simulink model "half_bridge"  (R2020a)
settings: Solver=VariableStepAuto  StartTime=0.0  StopTime=0.005  RelTol=1e-3
libraries: powerlib x25
settings Model: Creator=tomi_  LastModifiedBy=tomi_

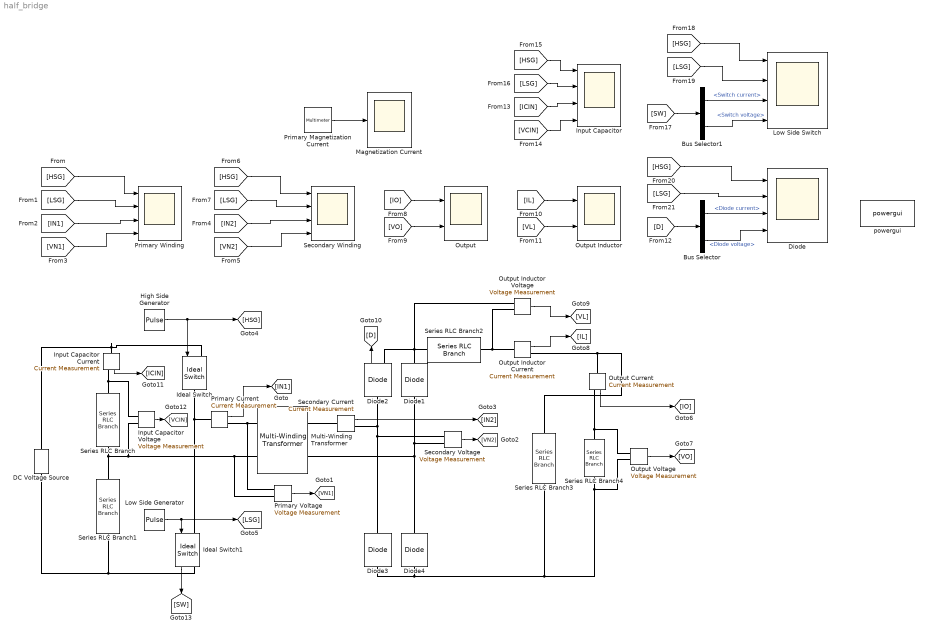
== system half_bridge ==
  Bus Selector : BusSelector  OutputSignals=Diode current,Diode voltage
  Bus Selector1 : BusSelector  OutputSignals=Switch current,Switch voltage
  DC Voltage Source : powerlib/Electrical Sources/DC Voltage Source  Amplitude=13.8  Measurements=None
  Diode : Scope  NumInputPorts=4
  Diode1 : powerlib/Power Electronics/Diode  Ron=0.0001  Lon=0  Vf=1  IC=0  UseSnubber=0  Rs=10e6  Cs=0  Measurements=off
  Diode2 : powerlib/Power Electronics/Diode  Ron=0.0001  Lon=0  Vf=1  IC=0  UseSnubber=0  Rs=10e6  Cs=0  Measurements=on
  Diode3 : powerlib/Power Electronics/Diode  Ron=0.0001  Lon=0  Vf=1  IC=0  UseSnubber=0  Rs=10e6  Cs=0  Measurements=off
  Diode4 : powerlib/Power Electronics/Diode  Ron=0.0001  Lon=0  Vf=1  IC=0  UseSnubber=0  Rs=10e6  Cs=0  Measurements=off
  High Side Generator : DiscretePulseGenerator  PulseType=Time based  Period=20e-6  PulseWidth=26.08
  Ideal Switch : powerlib/Power Electronics/Ideal Switch  Ron=0.0139  Lon=0  IC=0  Rs=10e6  Cs=inf  Measurements=off
  Ideal Switch1 : powerlib/Power Electronics/Ideal Switch  Ron=0.0139  Lon=0  IC=0  Rs=10e6  Cs=inf  Measurements=on
  Input Capacitor : Scope  NumInputPorts=4
  Input Capacitor Current : powerlib/Measurements/Current Measurement  PhasorSimulation=off  OutputType=Complex  PSBequivalent=0
  Input Capacitor Voltage : powerlib/Measurements/Voltage Measurement  PhasorSimulation=off  OutputType=Complex  PSBequivalent=0
  Low Side Generator : DiscretePulseGenerator  PulseType=Time based  Period=20e-6  PulseWidth=26.08  PhaseDelay=10e-6
  Low Side Switch : Scope  NumInputPorts=4
  Magnetization Current : Scope
  Multi-Winding Transformer : powerlib/Elements/Multi-Winding Transformer  LeftWindings=1  RightWindings=1  TappedWindings=no taps  NumberOfTaps=2  SetSaturation=off  Hysteresis=off  DataFile='hysteresis.mat'  Measurements=Flux and magnetization current ( Imag )  UNITS=SI  NominalPower=[ 75 100e3 ]  NominalVoltages=[ 6.9 604.9 ]  WindingResistances=[ 0 0 ]  WindingInductances=[0 0]  Rm=Inf  Lm=4.68e-5  Saturation=[0 0;0.27174 0.0010067;113.22 0.0012752]  BreakLoop=off  DiscreteSolver=Trapezoidal iterative  DataType=on  InitialFlux=0  TransfoNumber=1
      settings: SourceProductBaseCode=PS
  Output : Scope  NumInputPorts=2
  Output Current : powerlib/Measurements/Current Measurement  PhasorSimulation=off  OutputType=Complex  PSBequivalent=0
  Output Inductor : Scope  NumInputPorts=2
  Output Inductor Current : powerlib/Measurements/Current Measurement  PhasorSimulation=off  OutputType=Complex  PSBequivalent=0
  Output Inductor Voltage : powerlib/Measurements/Voltage Measurement  PhasorSimulation=off  OutputType=Complex  PSBequivalent=0
  Output Voltage : powerlib/Measurements/Voltage Measurement  PhasorSimulation=off  OutputType=Complex  PSBequivalent=0
  Primary Current : powerlib/Measurements/Current Measurement  PhasorSimulation=off  OutputType=Complex  PSBequivalent=0
  Primary Magnetization Current : powerlib/Measurements/Multimeter  PhasorSimulation=off  OutputType=Complex  sel=2  L=3  Gain=1  yselected={'Imag: Multi-Winding Transformer'};  PSBOutputType=1  PSBequivalent=0  AxesSetting=[0,0.1,-100,100]  Display=0  SavedBlockNames=-11
  Primary Voltage : powerlib/Measurements/Voltage Measurement  PhasorSimulation=off  OutputType=Complex  PSBequivalent=0
  Primary Winding : Scope  NumInputPorts=4
  Secondary Current : powerlib/Measurements/Current Measurement  PhasorSimulation=off  OutputType=Complex  PSBequivalent=0
  Secondary Voltage : powerlib/Measurements/Voltage Measurement  PhasorSimulation=off  OutputType=Complex  PSBequivalent=0
  Secondary Winding : Scope  NumInputPorts=4
  Series RLC Branch : powerlib/Elements/Series RLC Branch  LConnTagsString=__new0  RConnTagsString=__new0  BranchType=RC  Resistance=10e-3  Inductance=1e-3  SetiL0=off  InitialCurrent=0  Capacitance=680e-6  Setx0=off  InitialVoltage=0  Measurements=None
  Series RLC Branch1 : powerlib/Elements/Series RLC Branch  LConnTagsString=__new0  RConnTagsString=__new0  BranchType=RC  Resistance=10e-3  Inductance=1e-3  SetiL0=off  InitialCurrent=0  Capacitance=680e-6  Setx0=off  InitialVoltage=0  Measurements=None
  Series RLC Branch2 : powerlib/Elements/Series RLC Branch  LConnTagsString=__new0  RConnTagsString=__new0  BranchType=L  Resistance=1  Inductance=6.4e-3  SetiL0=off  InitialCurrent=0  Capacitance=1e-6  Setx0=off  InitialVoltage=0  Measurements=None
  Series RLC Branch3 : powerlib/Elements/Series RLC Branch  LConnTagsString=__new0  RConnTagsString=__new0  BranchType=RC  Resistance=100e-3  Inductance=1e-3  SetiL0=off  InitialCurrent=0  Capacitance=220e-9  Setx0=off  InitialVoltage=0  Measurements=None
  Series RLC Branch4 : powerlib/Elements/Series RLC Branch  LConnTagsString=__new0  RConnTagsString=__new0  BranchType=R  Resistance=1666  Inductance=1e-3  SetiL0=off  InitialCurrent=0  Capacitance=1e-6  Setx0=off  InitialVoltage=0  Measurements=None
  powergui : powerlib/powergui  Priority=1  SimulationMode=Continuous  SampleTime=100e-9  frequency=60  Iterations=50  frequencyindice=0  Pbase=100e6  ErrMax=1e-4  UnitsV=kV  UnitsW=MW  buscounter=0  FunctionMessages=off  echomessages=off  EnableUseOfTLC=off  CurrentSourceSwitches=off  DisableSnubberDevices=off  DisableRonSwitches=off  DisableVfSwitches=off  DisplayEquations=off  AutomaticDiscreteSolvers=off  SolverType=Tustin/Backward Euler (TBE)  Interpol=off  ExternalGateDelay=off  methode=off  Ts=100  x0status=blocks  SPID=on  SwTol=0  HookPort=off  NonlinearTolerance=1e-4  nMaxIteration=100  ContinueOnMaxIteration=off  RestoreLinks=warning  ResistiveCurrentMeasurement=off  Frange=[0:2:500]  Ylog=off  Xlog=on  ShowGrid=off  save=off  variable=ZData  structure=0  ZoomFFT=off  StartTime=0.0  cycles=1  DisplayStyle=1  fundamental=60  FreqAxis=off  MaxFrequency=1000  frequencyindicesteady=1  RmsSteady=1  display=off
  wires:
  High Side Generator/1 -> [HSG], Ideal Switch/1
  Low Side Generator/1 -> [LSG], Ideal Switch1/1
  Output Voltage/1 -> [VO]
  Secondary Voltage/1 -> [VN2]
  Primary Current/1 -> [IN1]
  Primary Voltage/1 -> [VN1]
  Secondary Current/1 -> [IN2]
  [HSG] -> Primary Winding/1
  [LSG] -> Primary Winding/2
  [IN1] -> Primary Winding/3
  [VN1] -> Primary Winding/4
  [LSG] -> Secondary Winding/2
  [VN2] -> Secondary Winding/4
  [IN2] -> Secondary Winding/3
  [HSG] -> Secondary Winding/1
  Output Current/1 -> [IO]
  [IO] -> Output/1
  [VO] -> Output/2
  Output Inductor Current/1 -> [IL]
  Output Inductor Voltage/1 -> [VL]
  [VL] -> Output Inductor/2
  [IL] -> Output Inductor/1
  Diode2/1 -> [D]
  [D] -> Bus Selector/1
  Bus Selector/1 -> Diode/3  "<Diode current>"
  Bus Selector/2 -> Diode/4  "<Diode voltage>"
  Input Capacitor Current/1 -> [ICIN]
  Input Capacitor Voltage/1 -> [VCIN]
  [LSG] -> Input Capacitor/2
  [ICIN] -> Input Capacitor/3
  [VCIN] -> Input Capacitor/4
  [HSG] -> Input Capacitor/1
  Ideal Switch1/1 -> [SW]
  Bus Selector1/2 -> Low Side Switch/4  "<Switch voltage>"
  Bus Selector1/1 -> Low Side Switch/3  "<Switch current>"
  [SW] -> Bus Selector1/1
  [LSG] -> Low Side Switch/2
  [HSG] -> Low Side Switch/1
  Primary Magnetization Current/1 -> Magnetization Current/1
  [LSG] -> Diode/2
  [HSG] -> Diode/1
  connections:
  Series RLC Branch/RConn1 -- Input Capacitor Voltage/LConn2 -- Multi-Winding Transformer/LConn2 -- Primary Voltage/LConn2 -- Series RLC Branch1/LConn1
  DC Voltage Source/RConn1 -- Ideal Switch/LConn1 -- Input Capacitor Current/LConn1
  Series RLC Branch1/RConn1 -- Ideal Switch1/RConn1 -- DC Voltage Source/LConn1
  Primary Current/LConn1 -- Ideal Switch1/LConn1 -- Ideal Switch/RConn1
  Secondary Voltage/LConn1 -- Diode3/RConn1 -- Diode2/LConn1 -- Secondary Current/RConn1
  Diode1/LConn1 -- Secondary Voltage/LConn2 -- Diode4/RConn1 -- Multi-Winding Transformer/RConn2
  Series RLC Branch2/LConn1 -- Diode1/RConn1 -- Diode2/RConn1 -- Output Inductor Voltage/LConn1
  Series RLC Branch3/LConn1 -- Output Inductor Current/RConn1 -- Output Current/LConn1
  Series RLC Branch3/RConn1 -- Output Voltage/LConn2 -- Series RLC Branch4/RConn1 -- Diode3/LConn1 -- Diode4/LConn1
  Primary Voltage/LConn1 -- Primary Current/RConn1 -- Multi-Winding Transformer/LConn1
  Secondary Current/LConn1 -- Multi-Winding Transformer/RConn1
  Series RLC Branch4/LConn1 -- Output Current/RConn1 -- Output Voltage/LConn1
  Output Inductor Current/LConn1 -- Output Inductor Voltage/LConn2 -- Series RLC Branch2/RConn1
  Series RLC Branch/LConn1 -- Input Capacitor Current/RConn1 -- Input Capacitor Voltage/LConn1
